simulink library "Lib_SlopA"  (R2021a)
settings: Solver=VariableStepAuto  StartTime=0.0  StopTime=10.0  RelTol=1e-3
libraries: simulink x1
settings Model: Creator=30610  LastModifiedBy=30610

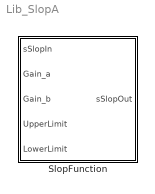
== system Lib_SlopA ==
  SlopFunction : Subsystem

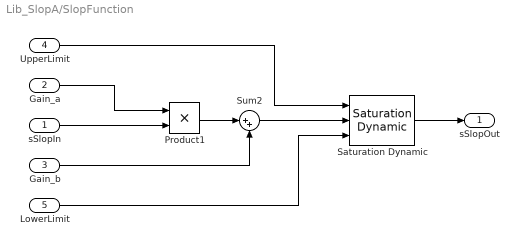
== system Lib_SlopA/SlopFunction ==
  sSlopIn : Inport  OutDataTypeStr=single
  Gain_a : Inport  Port=2  OutDataTypeStr=single
  Gain_b : Inport  Port=3  OutDataTypeStr=single
  UpperLimit : Inport  Port=4  OutDataTypeStr=single
  LowerLimit : Inport  Port=5  OutDataTypeStr=single
  Product1 : Product
  Saturation Dynamic : simulink/Discontinuities/Saturation Dynamic  OutMin=[]  OutMax=[]  OutDataTypeStr=Inherit: Same as second input  OutDataType=fixdt(1, 16)  OutScaling=2^-10  DoSatur=off
  Sum2 : Sum  Inputs=|++
  sSlopOut : Outport  OutDataTypeStr=single
  wires:
  sSlopIn/1 -> Product1/2
  Gain_b/1 -> Sum2/2
  Product1/1 -> Sum2/1
  Gain_a/1 -> Product1/1
  Saturation Dynamic/1 -> sSlopOut/1
  Sum2/1 -> Saturation Dynamic/2
  UpperLimit/1 -> Saturation Dynamic/1
  LowerLimit/1 -> Saturation Dynamic/3
